simulink model "QAM16_NDATED_DDPED_2023b"  (R2023b)
settings: Solver=ode45  StartTime=0  StopTime=3200  RelTol=1e-3  EnableMultiTasking=on
PreLoadFcn:
  | SNR=30;                          % Signal-to-noise ratio
  | M=16;                             % No. QAM symbols
  | m=4;                               % log2(M) bits/symbol
  | T =  0.1;                          % Symbol period
  | Tc = T/10;                       % Carrier period
  | deltaf = 3e-3*(1/T);          % Frequency error
  | Tr = T+100e-6*T;            % Receiver clock
  | alpha = 0.25;                   % Rolloff factor
  | 
  | b3 = [1/6 -1/2  1/2 -1/6];
  | b2 = [1/2 -1    1/2  0];
  | b1 = [1/3  1/2 -1    1/6];
  | b0 = [0    1    0    0];
  | 
  | warning off all
values from neighbouring files (symbols this model uses):
  seed = input('Enter the last five digits of your student ID: ')    [run_OFDM_2011b.m]    (also in run_OFDM_2024b.m; run_RAKE_Rayleigh_2021b.m = input('Enter your student ID: '); run_RAKE_Rayleigh_2024b.m = input('Enter your student ID: '))
undefined symbols (not defined in the file or in its folder): dfilt, doppler, gcbh, QAM, rcfiltgaincompat
libraries: dspobslib x7, commfilt2 x4, dspfdesign x3, commdigbbndam3 x3, commchan3 x2, commrandsrc2 x1
settings Model: Creator=professor  LastModifiedBy=14083
settings SolverCC: AlgebraicLoopSolver=TrustRegion
settings DataIOCC: LimitDataPoints=on  SaveFormat=Array  SignalLoggingSaveFormat=ModelDataLogs  ReturnWorkspaceOutputs=off
settings OptimizationCC: ExpressionDepthLimit=2147483647  InitFltsAndDblsToZero=on  LifeSpan=inf
settings DebuggingCC: AlgebraicLoopMsg=none  SaveWithParameterizedLinksMsg=none  UnderspecifiedInitializationDetection=Classic  MergeDetectMultiDrivingBlocksExec=none  SolverPrmCheckMsg=warning  MultiTaskDSMMsg=warning  MultiTaskCondExecSysMsg=none  FcnCallInpInsideContextMsg=warning  UnconnectedInputMsg=warning  UnconnectedOutputMsg=warning  UnconnectedLineMsg=warning  StateNameClashWarn=warning  SFUnexpectedBacktrackingDiag=warning  SFNoUnconditionalDefaultTransitionDiag=warning  SFExecutionAtInitializationDiag=none  ArithmeticOperatorsInVariantConditions=warning
settings HardwareCC: ProdBitPerPointer=32  ProdBitPerSizeT=32  ProdBitPerPtrDiffT=32  ProdLargestAtomicFloat=None  ProdIntDivRoundTo=Undefined  ProdEndianess=Unspecified  ProdWordSize=32  ProdHWDeviceType=32-bit Generic
settings ModelReferenceCC: EnableRefExpFcnMdlSchedulingChecks=on  PropagateSignalLabelsOutOfModel=off
settings SFSimCC: SimUseLocalCustomCode=off  CustomCodeUndefinedFunction=UseInterfaceOnly
settings RTWCC: RTWUseLocalCustomCode=off
settings CodeAppCC: StateflowObjectComments=on
settings GRTTargetCC: TargetFcnLib=ansi_tfl_tmw.mat  TargetLangStandard=C89/C90 (ANSI)  CombineOutputUpdateFcns=off  GRTInterface=on
settings ConfigComp: CovMetricSettings=dw  CovSaveCumulativeToWorkspaceVar=on  CovSaveSingleToWorkspaceVar=on  CovExternalEMLEnable=off

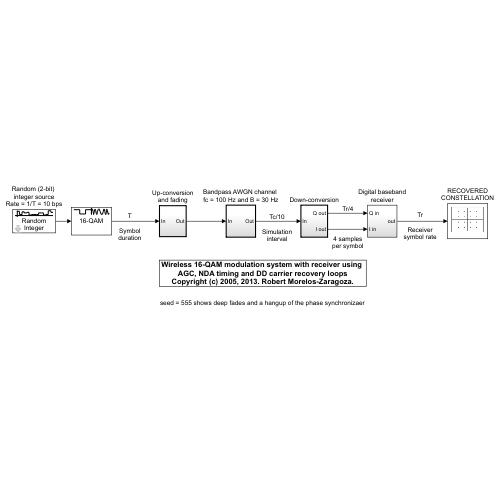
[thumbnail: Simulink's stored preview of the top-level diagram]
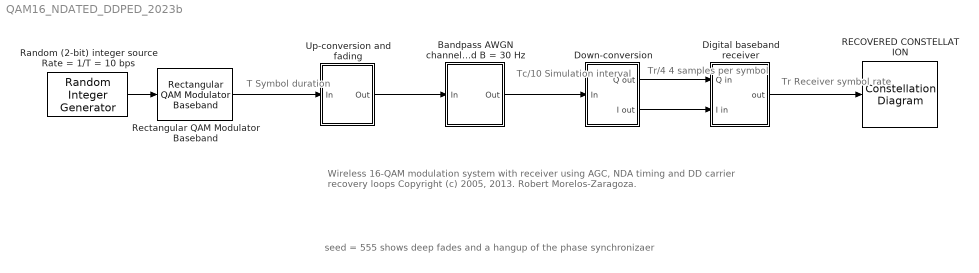
== system QAM16_NDATED_DDPED_2023b ==
  note: seed = 555 shows deep fades and a hangup of the phase synchronizaer
  note: Wireless 16-QAM modulation system with receiver using
      | AGC, NDA timing and DD carrier recovery loops
      | Copyright (c) 2005, 2013. Robert Morelos-Zaragoza.
  note: Tc/10
      |
      | Simulation
      | interval
  note: T
      |
      | Symbol
      | duration
  note: Tr/4
      |
      |
      |
      | 4 samples
      | per symbol
  note: Tr
      |
      | Receiver
      | symbol rate
  Bandpass AWGN channel fc = 100 Hz and B = 30 Hz : Subsystem  TreatAsAtomicUnit=on
  Digital baseband receiver : Subsystem
  Down-conversion : Subsystem  TreatAsAtomicUnit=on
  RECOVERED CONSTELLATION : ConstellationDiagram  Tag=ScatterPlot  WindowPosition=[323.000000,481.000000,326.000000,350.000000,]  Visible=on  ScopeFrameLocation=window  SymbolsToDisplaySource=Property  SymbolsToDisplay=150  ReferenceConstellation=16-QAM  Title=RECOVERED CONSTELLATION  XLimits=[-2.76,2.76]  YLimits=[-2.5 2.5]  DefaultConfigurationName=comm.scopes.ConstellationDiagramBlockCfg
  Random (2-bit) integer source Rate = 1/T = 10 bps : commrandsrc2/Random Integer Generator  mul=M  seed=seed  Ts=T  frameBased=off  sampPerFrame=1  orient=off  outDataType=double
  Rectangular QAM Modulator Baseband : commdigbbndam3/Rectangular QAM Modulator Baseband  M=M  InType=Integer  Enc=Gray  Mapping=[0:15]  PowType=Average Power  MinDist=2  AvgPow=1  PeakPow=1  Ph=0  outDtype=double  outWordLen=16  outUDDataType=sfix(16)  outFracLenMode=Best precision  outFracLen=15  outDataTypeStr=double  outLastDataTypeStr=double
  Up-conversion and fading : Subsystem  TreatAsAtomicUnit=on
  wires:
  Bandpass AWGN channel fc = 100 Hz and B = 30 Hz/1(Out) -> Down-conversion/1(In)
  Down-conversion/1(Q out) -> Digital baseband receiver/1(Q in)
  Down-conversion/2(I out) -> Digital baseband receiver/2(I in)
  Digital baseband receiver/1(out) -> RECOVERED CONSTELLATION/1
  Rectangular QAM Modulator Baseband/1 -> Up-conversion and fading/1(In)
  Random (2-bit) integer source Rate = 1/T = 10 bps/1 -> Rectangular QAM Modulator Baseband/1
  Up-conversion and fading/1(Out) -> Bandpass AWGN channel fc = 100 Hz and B = 30 Hz/1(In)

== system QAM16_NDATED_DDPED_2023b/Bandpass AWGN channel fc = 100 Hz and B = 30 Hz ==
  note: Bandpass AWGN channel
      |
      | Robert Morelos-Zaragoza
      | San Jose State University
      | Copyright (c) 2005
  In : Inport
  AWGN Channel : commchan3/AWGN Channel  LegacyMode=on  NoiseMethod="Signal to noise ratio  (SNR)"  noiseMode="Signal to noise ratio  (Eb/No)"  EbNo=SNR  EsNo=15  SNR=10  BitsPerSymbol=2  SignalPower=1  SamplesPerSymbol=1  SymbolPeriod=T/4  VarianceSource=Parameter  Variance=1  RandomStream=Global stream  Seed=13357  SimulateUsing=Code generation
  "Channel Hc(f) fc=100, B=30" : dspfdesign/Analog Filter Design  method=Chebyshev I  filttype=Bandpass  N=20  Wlo=2*pi*85  Whi=2*pi*115  Rp=0.5  Rs=30
  Tc/10 Simulation interval : ZeroOrderHold  SampleTime=Tc/10
  Out : Outport
  wires:
  "Channel Hc(f) fc=100, B=30"/1 -> Tc/10 Simulation interval/1
  AWGN Channel/1 -> Out/1
  In/1 -> "Channel Hc(f) fc=100, B=30"/1
  Tc/10 Simulation interval/1 -> AWGN Channel/1

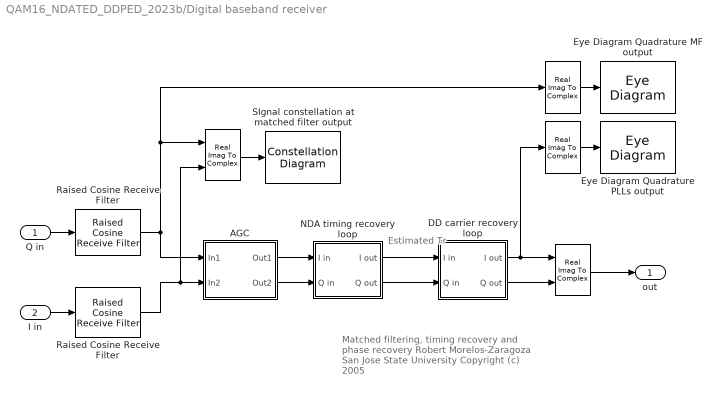
== system QAM16_NDATED_DDPED_2023b/Digital baseband receiver ==
  note: Estimated
      | Tr
  note: Matched filtering, timing recovery
      | and phase recovery
      |
      | Robert Morelos-Zaragoza
      | San Jose State University
      | Copyright (c) 2005
  Q in : Inport
  I in : Inport  Port=2
  " " : RealImagToComplex  Input=Real  SampleTime=Tr/4
  "    " : RealImagToComplex  SampleTime=Tr/4
  "       " : RealImagToComplex  Input=Real  SampleTime=Tr/4
  "           " : RealImagToComplex  SampleTime=Tr
  AGC : Subsystem  TreatAsAtomicUnit=on
  DD carrier recovery loop : Subsystem
  Eye Diagram Quadrature MF output : EyeDiagram  Tag=EyeDiagram
  Eye Diagram Quadrature PLLs output : EyeDiagram  Tag=EyeDiagram
  NDA timing recovery loop : Subsystem
  Raised Cosine Receive Filter : commfilt2/Raised Cosine Receive Filter  filtType=Square root  R=alpha  filtSpan=2*(4)  N=4  downFactor=1  downOffset=0  filterGain=(1/2)*rcfiltgaincompat(gcbh)  InputProcessing=Columns as channels (frame based)  RateOptions=Enforce single-rate processing  framing=Mute  checkCoeff=off  variableName=rcRxFilt  currentFiltSpan=2*(4)  D=4  inputOffset=0  sampMode=Mute  saveAsFlag=0  rateMode=Downsampling  checkGain=User-specified  launchFVT=off  roundingMode=Floor  overflowMode=off  coeffDataTypeStr=Inherit: Same word length as input  coeffMin=[]  coeffMax=[]  coeffLastDataTypeStr=Inherit: Same word length as input  accumDataTypeStr=Inherit: Same as product output  accumLastDataTypeStr=Inherit: Same as product output  outputDataTypeStr=Inherit: Same as accumulator  outputMin=[]  outputMax=[]  outputLastDataTypeStr=Inherit: Same as accumulator
  "Raised Cosine Receive Filter " : commfilt2/Raised Cosine Receive Filter  filtType=Square root  R=alpha  filtSpan=2*(4)  N=4  downFactor=1  downOffset=0  filterGain=(1/2)*rcfiltgaincompat(gcbh)  InputProcessing=Columns as channels (frame based)  RateOptions=Enforce single-rate processing  framing=Mute  checkCoeff=off  variableName=rcRxFilt1  currentFiltSpan=2*(4)  D=4  inputOffset=0  sampMode=Mute  saveAsFlag=0  rateMode=Downsampling  checkGain=User-specified  launchFVT=off  roundingMode=Floor  overflowMode=off  coeffDataTypeStr=Inherit: Same word length as input  coeffMin=[]  coeffMax=[]  coeffLastDataTypeStr=Inherit: Same word length as input  accumDataTypeStr=Inherit: Same as product output  accumLastDataTypeStr=Inherit: Same as product output  outputDataTypeStr=Inherit: Same as accumulator  outputMin=[]  outputMax=[]  outputLastDataTypeStr=Inherit: Same as accumulator
  SIgnal constellation at matched filter output : ConstellationDiagram  Tag=ScatterPlot  WindowPosition=[-1.000000,481.000000,322.000000,351.000000,]  Visible=on  ScopeFrameLocation=window  SamplesPerSymbol=4  SampleOffset=1  SymbolsToDisplaySource=Property  SymbolsToDisplay=150  ReferenceConstellation=16-QAM  Title=MF OUTPUT CONSTELLATION  XLimits=[-2.71,2.71]  YLimits=[-2.5 2.5]  DefaultConfigurationName=comm.scopes.ConstellationDiagramBlockCfg
  out : Outport
  wires:
  Q in/1 -> Raised Cosine Receive Filter/1
  I in/1 -> "Raised Cosine Receive Filter "/1
  Raised Cosine Receive Filter/1 -> "    "/1, " "/1, AGC/1(In1)
  "    "/1 -> SIgnal constellation at matched filter output/1
  DD carrier recovery loop/1(I out) -> "           "/1, "       "/1
  DD carrier recovery loop/2(Q out) -> "           "/2
  "           "/1 -> out/1
  NDA timing recovery loop/1(I out) -> DD carrier recovery loop/1(I in)
  NDA timing recovery loop/2(Q out) -> DD carrier recovery loop/2(Q in)
  " "/1 -> Eye Diagram Quadrature MF output/1
  "       "/1 -> Eye Diagram Quadrature PLLs output/1
  "Raised Cosine Receive Filter "/1 -> "    "/2, AGC/2(In2)
  AGC/1(Out1) -> NDA timing recovery loop/1(I in)
  AGC/2(Out2) -> NDA timing recovery loop/2(Q in)

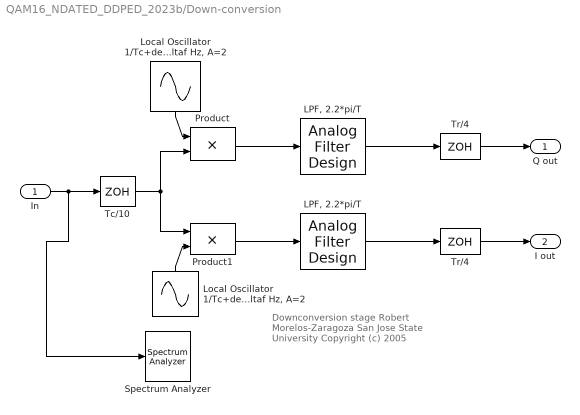
== system QAM16_NDATED_DDPED_2023b/Down-conversion ==
  note: Downconversion stage
      |
      | Robert Morelos-Zaragoza
      | San Jose State University
      | Copyright (c) 2005
  In : Inport
  " LPF, 2.2*pi/T " : dspfdesign/Analog Filter Design  method=Butterworth  filttype=Lowpass  N=8  Wlo=2.2*pi/T  Whi=80  Rp=2  Rs=40
  "LPF, 2.2*pi/T" : dspfdesign/Analog Filter Design  method=Butterworth  filttype=Lowpass  N=8  Wlo=2.2*pi/T  Whi=80  Rp=2  Rs=40
  "Local Oscillator 1/Tc+deltaf Hz, A=2 " : Sin  Amplitude=2  Frequency=2*pi/Tc+deltaf  SampleTime=Tc/10
  "Local Oscillator 1/Tc+deltaf Hz, A=2    " : Sin  Amplitude=2  Frequency=2*pi/Tc+deltaf  Phase=pi/2  SampleTime=Tc/10
  Product : Product  InputSameDT=on  SaturateOnIntegerOverflow=on  OutDataTypeStr=Inherit: Same as first input
  Product1 : Product  InputSameDT=on  SaturateOnIntegerOverflow=on  OutDataTypeStr=Inherit: Same as first input
  Spectrum Analyzer : SpectrumAnalyzer  WindowPosition=[1055.000000,511.000000,477.000000,319.000000,]  Visible=on  ScopeFrameLocation=window  AxesScaling=Manual  Span=1000  StartFrequency=-500  StopFrequency=500  YLimits=[-30,30]
  Tc/10 : ZeroOrderHold  SampleTime=Tc/10
  Tr/4 : ZeroOrderHold  SampleTime=Tr/4
  "Tr/4 " : ZeroOrderHold  SampleTime=Tr/4
  Q out : Outport
  I out : Outport  Port=2
  wires:
  "Local Oscillator 1/Tc+deltaf Hz, A=2    "/1 -> Product1/2
  "LPF, 2.2*pi/T"/1 -> Tr/4/1
  "Local Oscillator 1/Tc+deltaf Hz, A=2 "/1 -> Product/1
  Product/1 -> "LPF, 2.2*pi/T"/1
  " LPF, 2.2*pi/T "/1 -> "Tr/4 "/1
  Product1/1 -> " LPF, 2.2*pi/T "/1
  In/1 -> Spectrum Analyzer/1, Tc/10/1
  Tr/4/1 -> Q out/1
  "Tr/4 "/1 -> I out/1
  Tc/10/1 -> Product/2, Product1/1

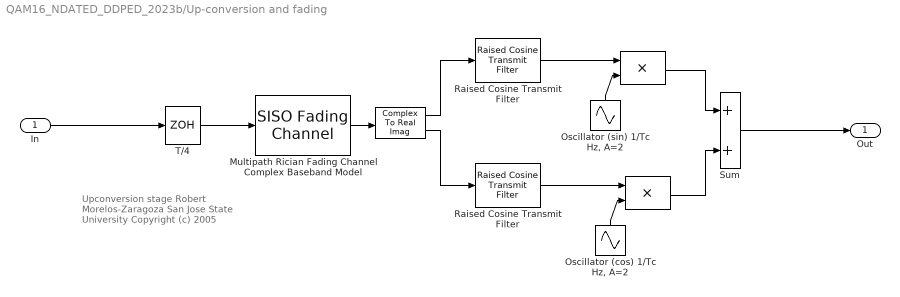
== system QAM16_NDATED_DDPED_2023b/Up-conversion and fading ==
  note: Upconversion stage
      |
      | Robert Morelos-Zaragoza
      | San Jose State University
      | Copyright (c) 2005
  In : Inport
  " " : ComplexToRealImag
  "  " : Product  InputSameDT=on  SaturateOnIntegerOverflow=on  OutDataTypeStr=Inherit: Same as first input
  "   " : Product  InputSameDT=on  SaturateOnIntegerOverflow=on  OutDataTypeStr=Inherit: Same as first input
  Multipath Rician Fading Channel Complex Baseband Model : commchan3/SISO Fading Channel  InheritSampleRate=on  SampleRate=1  PathDelays=0  AveragePathGains=-3  NormalizePathGains=on  FadingDistribution=Rician  KFactor=1  DirectPathDopplerShift=.001  DirectPathInitialPhase=0  MaximumDopplerShift=7e-5  DopplerSpectrum=doppler('Jakes')  RandomStream=mt19937ar with seed  Seed=mod(seed,100)  PathGainsOutputPort=off  ChannelFilterDelayOutputPort=off  SimulateUsing=Interpreted execution  Visualization=Off  PathsForDopplerDisplay=1  SamplesToDisplay=25%
  "Oscillator (cos) 1/Tc Hz, A=2" : Sin  Amplitude=2  Frequency=2*pi/Tc  Phase=pi/2  SampleTime=0
  "Oscillator (sin) 1/Tc Hz, A=2 " : Sin  Amplitude=2  Frequency=2*pi/Tc  SampleTime=0
  Raised Cosine Transmit Filter : commfilt2/Raised Cosine Transmit Filter  filtType=Square root  R=alpha  filtSpan=2*(4)  N=4  filterGain=rcfiltgaincompat(gcbh)  InputProcessing=Columns as channels (frame based)  RateOptions=Allow multirate processing  framing=Mute  checkCoeff=off  variableName=rcTxFilt  checkGain=Normalized  sampMode=Mute  saveAsFlag=0  currentFiltSpan=2*(4)  D=4  launchFVT=off  roundingMode=Floor  overflowMode=off  coeffDataTypeStr=Inherit: Same word length as input  coeffMin=[]  coeffMax=[]  coeffLastDataTypeStr=Inherit: Same word length as input  outputDataTypeStr=Inherit: Same as accumulator  outputMin=[]  outputMax=[]  outputLastDataTypeStr=Inherit: Same as accumulator
  "Raised Cosine Transmit Filter " : commfilt2/Raised Cosine Transmit Filter  filtType=Square root  R=alpha  filtSpan=2*(4)  N=4  filterGain=rcfiltgaincompat(gcbh)  InputProcessing=Columns as channels (frame based)  RateOptions=Allow multirate processing  framing=Mute  checkCoeff=off  variableName=rcTxFilt1  checkGain=Normalized  sampMode=Mute  saveAsFlag=0  currentFiltSpan=2*(4)  D=4  launchFVT=off  roundingMode=Floor  overflowMode=off  coeffDataTypeStr=Inherit: Same word length as input  coeffMin=[]  coeffMax=[]  coeffLastDataTypeStr=Inherit: Same word length as input  outputDataTypeStr=Inherit: Same as accumulator  outputMin=[]  outputMax=[]  outputLastDataTypeStr=Inherit: Same as accumulator
  Sum : Sum  InputSameDT=on  SaturateOnIntegerOverflow=on  OutDataTypeStr=Inherit: Same as first input
  T/4 : ZeroOrderHold  SampleTime=T/4
  Out : Outport
  wires:
  T/4/1 -> Multipath Rician Fading Channel Complex Baseband Model/1
  In/1 -> T/4/1
  Raised Cosine Transmit Filter/1 -> "  "/1
  "Raised Cosine Transmit Filter "/1 -> "   "/1
  "Oscillator (sin) 1/Tc Hz, A=2 "/1 -> "  "/2
  "Oscillator (cos) 1/Tc Hz, A=2"/1 -> "   "/2
  "  "/1 -> Sum/1
  "   "/1 -> Sum/2
  Sum/1 -> Out/1
  " "/1 -> Raised Cosine Transmit Filter/1
  " "/2 -> "Raised Cosine Transmit Filter "/1
  Multipath Rician Fading Channel Complex Baseband Model/1 -> " "/1

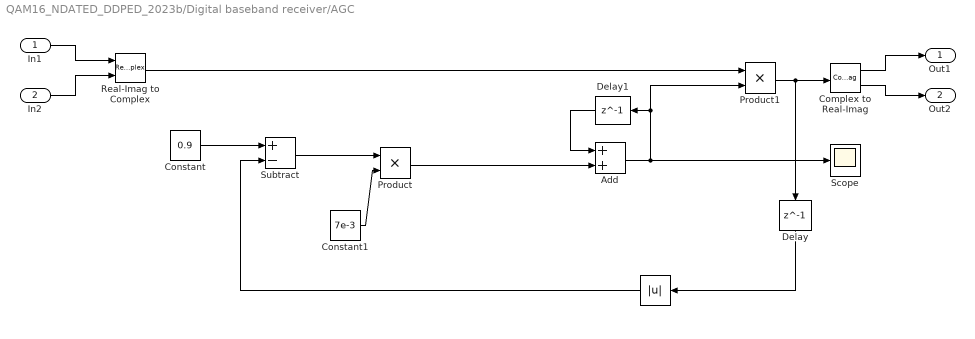
== system QAM16_NDATED_DDPED_2023b/Digital baseband receiver/AGC ==
  In1 : Inport
  In2 : Inport  Port=2
  " " : Abs  SaturateOnIntegerOverflow=off
  Add : Sum
  Complex to Real-Imag : ComplexToRealImag
  Constant : Constant  Value=0.9
  Constant1 : Constant  Value=7e-3
  Delay : Delay  DelayLength=1  InitialCondition=0  InputProcessing=Columns as channels (frame based)
  Delay1 : Delay  DelayLength=1  InitialCondition=1  InputProcessing=Columns as channels (frame based)
  Product : Product  RndMeth=Zero
  Product1 : Product  RndMeth=Zero
  Real-Imag to Complex : RealImagToComplex
  Scope : Scope
  Subtract : Sum  Inputs=+-
  Out1 : Outport
  Out2 : Outport  Port=2
  wires:
  Subtract/1 -> Product/1
  Constant1/1 -> Product/2
  In1/1 -> Real-Imag to Complex/1
  In2/1 -> Real-Imag to Complex/2
  Real-Imag to Complex/1 -> Product1/1
  Complex to Real-Imag/1 -> Out1/1
  Complex to Real-Imag/2 -> Out2/1
  Product1/1 -> Delay/1, Complex to Real-Imag/1
  Delay/1 -> " "/1
  Product/1 -> Add/2
  Add/1 -> Scope/1, Product1/2, Delay1/1
  Delay1/1 -> Add/1
  Constant/1 -> Subtract/1
  " "/1 -> Subtract/2

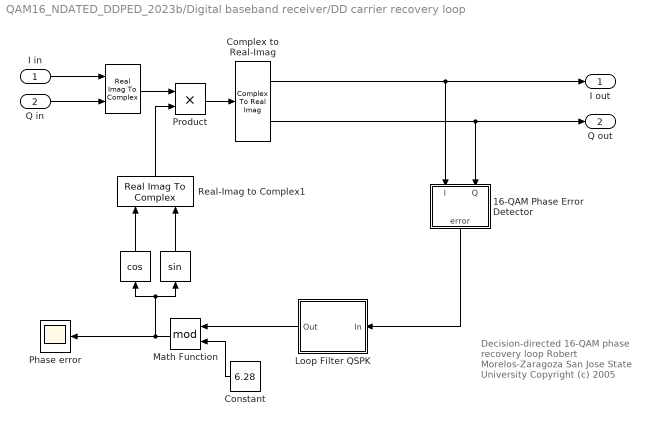
== system QAM16_NDATED_DDPED_2023b/Digital baseband receiver/DD carrier recovery loop ==
  note: Decision-directed 16-QAM
      | phase recovery loop
      |
      | Robert Morelos-Zaragoza
      | San Jose State University
      | Copyright (c) 2005
  I in : Inport
  Q in : Inport  Port=2
  " " : Trigonometry  OutputSignalType=real
  "   " : Trigonometry  Operator=cos  OutputSignalType=real
  "     " : RealImagToComplex  SampleTime=Tr
  "  16-QAM Phase Error Detector" : Subsystem
  Complex to Real-Imag : ComplexToRealImag
  Constant : Constant  Value=6.28  SampleTime=Tr
  Loop Filter QSPK : Subsystem
  Math Function : Math  Operator=mod  SignedPower=on  OutputSignalType=real  SampleTime=Tr
  Phase error : Scope
  Product : Product  InputSameDT=on  OutDataTypeStr=Inherit: Same as first input
  Real-Imag to Complex1 : RealImagToComplex
  I out : Outport
  Q out : Outport  Port=2
  wires:
  Real-Imag to Complex1/1 -> Product/2
  "   "/1 -> Real-Imag to Complex1/1
  " "/1 -> Real-Imag to Complex1/2
  Product/1 -> Complex to Real-Imag/1
  Complex to Real-Imag/1 -> I out/1, "  16-QAM Phase Error Detector"/1(I)
  Complex to Real-Imag/2 -> Q out/1, "  16-QAM Phase Error Detector"/2(Q)
  Loop Filter QSPK/1(Out) -> Math Function/1
  Constant/1 -> Math Function/2
  Math Function/1 -> " "/1, "   "/1, Phase error/1
  I in/1 -> "     "/1
  Q in/1 -> "     "/2
  "     "/1 -> Product/1
  "  16-QAM Phase Error Detector"/1(error) -> Loop Filter QSPK/1(In)

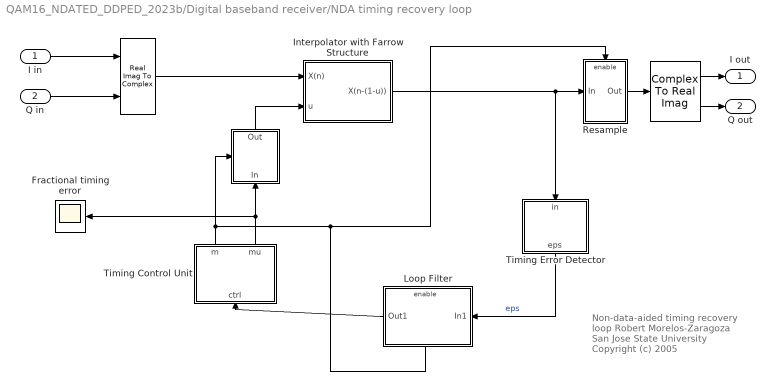
== system QAM16_NDATED_DDPED_2023b/Digital baseband receiver/NDA timing recovery loop ==
  note: Non-data-aided timing
      | recovery loop
      |
      | Robert Morelos-Zaragoza
      | San Jose State University
      | Copyright (c) 2005
  I in : Inport
  Q in : Inport  Port=2
  " " : ComplexToRealImag
  "     " : RealImagToComplex  SampleTime=Tr/4
  "         " : Subsystem  TreatAsAtomicUnit=on
  "  Timing Error Detector " : Subsystem
  Fractional timing error : Scope
  "Interpolator with Farrow Structure " : Subsystem
  "Loop Filter " : Subsystem  TreatAsAtomicUnit=on
  Resample : Subsystem  TreatAsAtomicUnit=on
  "Timing Control Unit   " : Subsystem
  I out : Outport
  Q out : Outport  Port=2
  wires:
  I in/1 -> "     "/1
  Q in/1 -> "     "/2
  "Interpolator with Farrow Structure "/1(X(n-(1-u))) -> Resample/1(In), "  Timing Error Detector "/1(in)
  "     "/1 -> "Interpolator with Farrow Structure "/1(X(n))
  "  Timing Error Detector "/1(eps) -> "Loop Filter "/1(In1)  "eps"
  " "/1 -> I out/1
  " "/2 -> Q out/1
  Resample/1(Out) -> " "/1
  "Loop Filter "/1(Out1) -> "Timing Control Unit   "/1(ctrl)
  "Timing Control Unit   "/2(mu) -> "         "/1(In), Fractional timing error/1
  "         "/1(Out) -> "Interpolator with Farrow Structure "/2(u)
  "Timing Control Unit   "/1(m) -> "         "/Enable, Resample/Enable, "Loop Filter "/Enable

== system QAM16_NDATED_DDPED_2023b/Digital baseband receiver/DD carrier recovery loop/  16-QAM Phase Error Detector ==
  I : Inport
  Q : Inport  Port=2
  Complex to Real-Imag : ComplexToRealImag  Output=Imag
  Math Function : Math  Operator=hermitian  SignedPower=on
  Product : Product  InputSameDT=on  RndMeth=Zero  SaturateOnIntegerOverflow=on  OutDataTypeStr=Inherit: Same as first input
  Real-Imag to Complex : RealImagToComplex
  Rectangular QAM Demodulator Baseband : commdigbbndam3/Rectangular QAM Demodulator Baseband  M=M  OutType=Integer  DecType=Hard decision  VarSource=Dialog  Variance=1  Dec=Gray  Mapping=[0:15]  PowType=Average Power  MinDist=2  AvgPow=1  PeakPow=1  Ph=0  outDtype1=Inherit via internal rule  outDtype2=Inherit via internal rule  derotateFactorWordLen=16  derotateFactorDataTypeStr=Inherit: Same word length as input  derotateFactorLastDataTypeStr=Inherit: Same word length as input  denormFactorWordLen=16  denormFactorDataTypeStr=Inherit: Same word length as input  denormFactorLastDataTypeStr=Inherit: Same word length as input  prodOutWordLen=32  prodOutOverflowMode=Wrap  prodOutRoundingMode=Floor  prodOutOvFlMode=off  prodOutOvFlModeLastStrValue=off  sumWordLen=32
  Rectangular QAM Modulator Baseband : commdigbbndam3/Rectangular QAM Modulator Baseband  M=M  InType=Integer  Enc=Gray  Mapping=[0:15]  PowType=Average Power  MinDist=2  AvgPow=1  PeakPow=1  Ph=0  outDtype=double  outWordLen=16  outUDDataType=sfix(16)  outFracLenMode=Best precision  outFracLen=15  outDataTypeStr=double  outLastDataTypeStr=double
  error : Outport
  wires:
  Rectangular QAM Demodulator Baseband/1 -> Rectangular QAM Modulator Baseband/1
  Real-Imag to Complex/1 -> Rectangular QAM Demodulator Baseband/1, Product/1
  I/1 -> Real-Imag to Complex/1
  Q/1 -> Real-Imag to Complex/2
  Product/1 -> Complex to Real-Imag/1
  Complex to Real-Imag/1 -> error/1
  Rectangular QAM Modulator Baseband/1 -> Math Function/1
  Math Function/1 -> Product/2

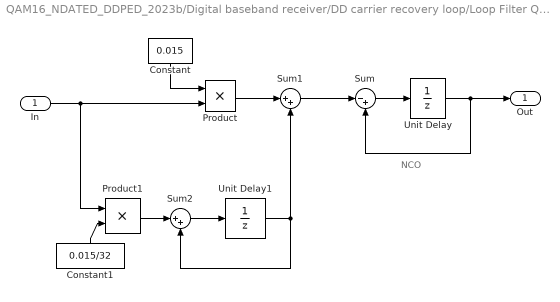
== system QAM16_NDATED_DDPED_2023b/Digital baseband receiver/DD carrier recovery loop/Loop Filter QSPK ==
  note: NCO
  In : Inport
  Constant : Constant  Value=0.015  SampleTime=Tr
  Constant1 : Constant  Value=0.015/32  SampleTime=Tr
  Product : Product  InputSameDT=on  SaturateOnIntegerOverflow=on  SampleTime=Tr  OutDataTypeStr=Inherit: Same as first input
  Product1 : Product  InputSameDT=on  SaturateOnIntegerOverflow=on  SampleTime=Tr  OutDataTypeStr=Inherit: Same as first input
  Sum : Sum  Inputs=|-+  InputSameDT=on  SaturateOnIntegerOverflow=on  OutDataTypeStr=Inherit: Same as first input
  Sum1 : Sum  Inputs=|++  InputSameDT=on  SaturateOnIntegerOverflow=on  OutDataTypeStr=Inherit: Same as first input
  Sum2 : Sum  Inputs=|++  InputSameDT=on  SaturateOnIntegerOverflow=on  OutDataTypeStr=Inherit: Same as first input
  Unit Delay : UnitDelay  SampleTime=Tr  HasFrameUpgradeWarning=on
  Unit Delay1 : UnitDelay  SampleTime=Tr  HasFrameUpgradeWarning=on
  Out : Outport
  wires:
  Product/1 -> Sum1/1
  Constant1/1 -> Product1/2
  Sum/1 -> Unit Delay/1
  Unit Delay/1 -> Out/1, Sum/2
  Constant/1 -> Product/1
  In/1 -> Product/2, Product1/1
  Product1/1 -> Sum2/1
  Sum2/1 -> Unit Delay1/1
  Unit Delay1/1 -> Sum1/2, Sum2/2
  Sum1/1 -> Sum/1

== system QAM16_NDATED_DDPED_2023b/Digital baseband receiver/NDA timing recovery loop/          ==
  In : Inport
  Enable : EnablePort
  Out : Outport
  wires:
  In/1 -> Out/1

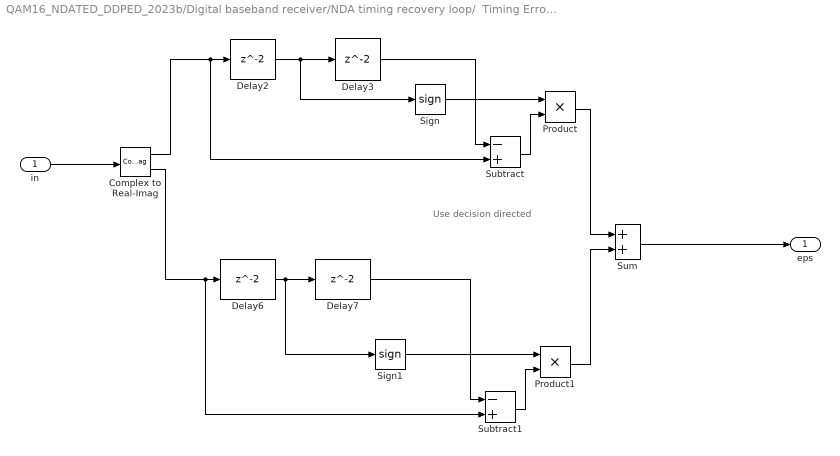
== system QAM16_NDATED_DDPED_2023b/Digital baseband receiver/NDA timing recovery loop/  Timing Error Detector  ==
  note: Use decision directed
  in : Inport
  Complex to Real-Imag : ComplexToRealImag
  Delay{2..3,6..7} (4 alike) : Delay  InitialCondition=0  InputProcessing=Columns as channels (frame based)
  Product : Product  RndMeth=Zero
  Product1 : Product  RndMeth=Zero
  Sign : Signum
  Sign1 : Signum
  Subtract : Sum  Inputs=-+
  Subtract1 : Sum  Inputs=-+
  Sum : Sum
  eps : Outport
  wires:
  Delay3/1 -> Subtract/1
  Delay7/1 -> Subtract1/1
  in/1 -> Complex to Real-Imag/1
  Complex to Real-Imag/1 -> Delay2/1, Subtract/2
  Complex to Real-Imag/2 -> Delay6/1, Subtract1/2
  Sum/1 -> eps/1
  Subtract1/1 -> Product1/2
  Product1/1 -> Sum/2
  Subtract/1 -> Product/2
  Product/1 -> Sum/1
  Delay2/1 -> Delay3/1, Sign/1
  Delay6/1 -> Delay7/1, Sign1/1
  Sign/1 -> Product/1
  Sign1/1 -> Product1/1

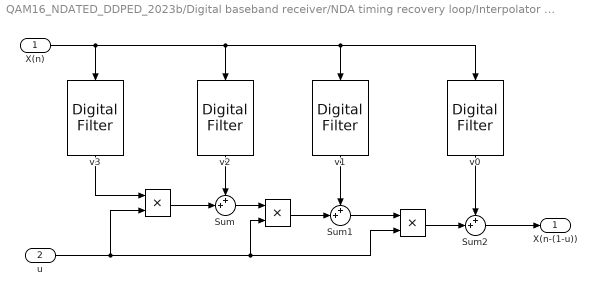
== system QAM16_NDATED_DDPED_2023b/Digital baseband receiver/NDA timing recovery loop/Interpolator with Farrow Structure  ==
  X(n) : Inport
  u : Inport  Port=2
  " " : Product  SaturateOnIntegerOverflow=on  OutDataTypeStr=Inherit: Same as first input
  "  " : Product  SaturateOnIntegerOverflow=on  OutDataTypeStr=Inherit: Same as first input
  "   " : Product  SaturateOnIntegerOverflow=on  OutDataTypeStr=Inherit: Same as first input
  Sum : Sum  Inputs=++|  SaturateOnIntegerOverflow=on
  Sum1 : Sum  Inputs=++|  SaturateOnIntegerOverflow=on
  Sum2 : Sum  Inputs=++|  SaturateOnIntegerOverflow=on
  v0 : dspobslib/Digital Filter  TypePopup=FIR (all zeros)  IIRFiltStruct=Direct form II transposed  AllPoleFiltStruct=Direct form  FIRFiltStruct=Direct form  CoeffSource=Specify via dialog  NumCoeffs=b0  DenCoeffs=[1 0.1]  BiQuadCoeffs=[1 0.3 0.4 1 0.1 0.2]  LatticeCoeffs=[0.2 0.4]  denIgnore=on  FiltPerSampPopup=One filter per frame  IC=0  ICnum=0  ICden=0  roundingMode=Floor  overflowMode=off  ScaleValues=1  scaleValueFracLength=14  stageInFracLength=15  stageOutFracLength=15  FilterSource=Specify via dialog  dfiltObjectName=dfilt.dffir([1 2 1])  InputProcessing=Columns as channels (frame based)
  v1 : dspobslib/Digital Filter  TypePopup=FIR (all zeros)  IIRFiltStruct=Direct form II transposed  AllPoleFiltStruct=Direct form  FIRFiltStruct=Direct form  CoeffSource=Specify via dialog  NumCoeffs=b1  DenCoeffs=[1 0.1]  BiQuadCoeffs=[1 0.3 0.4 1 0.1 0.2]  LatticeCoeffs=[0.2 0.4]  denIgnore=on  FiltPerSampPopup=One filter per frame  IC=0  ICnum=0  ICden=0  roundingMode=Floor  overflowMode=off  ScaleValues=1  scaleValueFracLength=14  stageInFracLength=15  stageOutFracLength=15  FilterSource=Specify via dialog  dfiltObjectName=dfilt.dffir([1 2 1])  InputProcessing=Columns as channels (frame based)
  v2 : dspobslib/Digital Filter  TypePopup=FIR (all zeros)  IIRFiltStruct=Direct form II transposed  AllPoleFiltStruct=Direct form  FIRFiltStruct=Direct form  CoeffSource=Specify via dialog  NumCoeffs=b2  DenCoeffs=[1 0.1]  BiQuadCoeffs=[1 0.3 0.4 1 0.1 0.2]  LatticeCoeffs=[0.2 0.4]  denIgnore=on  FiltPerSampPopup=One filter per frame  IC=0  ICnum=0  ICden=0  roundingMode=Floor  overflowMode=off  ScaleValues=1  scaleValueFracLength=14  stageInFracLength=15  stageOutFracLength=15  FilterSource=Specify via dialog  dfiltObjectName=dfilt.dffir([1 2 1])  InputProcessing=Columns as channels (frame based)
  v3 : dspobslib/Digital Filter  TypePopup=FIR (all zeros)  IIRFiltStruct=Direct form II transposed  AllPoleFiltStruct=Direct form  FIRFiltStruct=Direct form  CoeffSource=Specify via dialog  NumCoeffs=b3  DenCoeffs=[1 0.1]  BiQuadCoeffs=[1 0.3 0.4 1 0.1 0.2]  LatticeCoeffs=[0.2 0.4]  denIgnore=on  FiltPerSampPopup=One filter per frame  IC=0  ICnum=0  ICden=0  roundingMode=Floor  overflowMode=off  ScaleValues=1  scaleValueFracLength=14  stageInFracLength=15  stageOutFracLength=15  FilterSource=Specify via dialog  dfiltObjectName=dfilt.dffir([1 2 1])  InputProcessing=Columns as channels (frame based)
  X(n-(1-u)) : Outport
  wires:
  Sum2/1 -> X(n-(1-u))/1
  u/1 -> "   "/2, "  "/2, " "/2
  X(n)/1 -> v3/1, v2/1, v1/1, v0/1
  v0/1 -> Sum2/1
  v1/1 -> Sum1/1
  v2/1 -> Sum/1
  v3/1 -> " "/1
  " "/1 -> Sum/2
  Sum/1 -> "  "/1
  "  "/1 -> Sum1/2
  Sum1/1 -> "   "/1
  "   "/1 -> Sum2/2

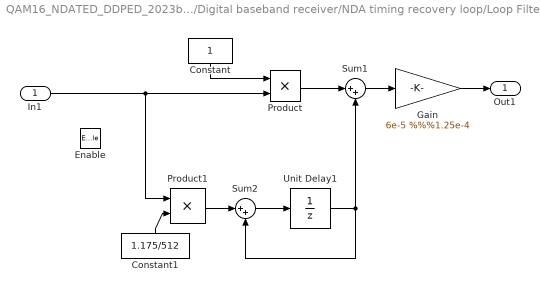
== system QAM16_NDATED_DDPED_2023b/Digital baseband receiver/NDA timing recovery loop/Loop Filter  ==
  In1 : Inport
  Enable : EnablePort
  Constant : Constant  SampleTime=Tr/4
  Constant1 : Constant  Value=1.175/512  SampleTime=Tr/4
  Gain : Gain  Gain=6e-5 %%%1.25e-4
  Product : Product  InputSameDT=on  SaturateOnIntegerOverflow=on  OutDataTypeStr=Inherit: Same as first input
  Product1 : Product  InputSameDT=on  SaturateOnIntegerOverflow=on  OutDataTypeStr=Inherit: Same as first input
  Sum1 : Sum  Inputs=|++  InputSameDT=on  SaturateOnIntegerOverflow=on  OutDataTypeStr=Inherit: Same as first input
  Sum2 : Sum  Inputs=|++  InputSameDT=on  SaturateOnIntegerOverflow=on  OutDataTypeStr=Inherit: Same as first input
  Unit Delay1 : UnitDelay  SampleTime=-1  HasFrameUpgradeWarning=on
  Out1 : Outport
  wires:
  Product/1 -> Sum1/1
  Constant1/1 -> Product1/2
  Constant/1 -> Product/1
  In1/1 -> Product/2, Product1/1
  Product1/1 -> Sum2/1
  Sum2/1 -> Unit Delay1/1
  Unit Delay1/1 -> Sum1/2, Sum2/2
  Sum1/1 -> Gain/1
  Gain/1 -> Out1/1

== system QAM16_NDATED_DDPED_2023b/Digital baseband receiver/NDA timing recovery loop/Resample ==
  In : Inport
  Enable : EnablePort
  Out : Outport
  wires:
  In/1 -> Out/1

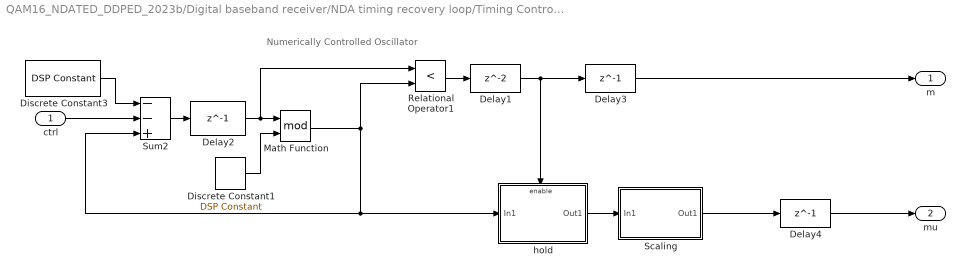
== system QAM16_NDATED_DDPED_2023b/Digital baseband receiver/NDA timing recovery loop/Timing Control Unit    ==
  note: Numerically Controlled Oscillator
  ctrl : Inport
  Delay1 : Delay  InitialCondition=0  InputProcessing=Columns as channels (frame based)
  Delay2 : Delay  DelayLength=1  InitialCondition=0  InputProcessing=Columns as channels (frame based)
  Delay3 : Delay  DelayLength=1  InitialCondition=0  InputProcessing=Columns as channels (frame based)
  Delay4 : Delay  DelayLength=1  InitialCondition=0  InputProcessing=Columns as channels (frame based)
  Discrete Constant1 : dspobslib/DSP Constant  Value=1  SampleMode=Discrete  discreteOutput=Sample-based (interpret vectors as 1-D)  continuousOutput=Sample-based  sampTime=Tr/4  framePeriod=Tr/4  dataType=Inherit via back propagation  isSigned=on  wordLen=16  udDataType=sfix(16)  fracBitsMode=Best precision  numFracBits=15  InterpretAs1D=on  Ts=Tr/4  FramebasedOutput=off
      settings: additionalParams=on
  Discrete Constant3 : dspobslib/DSP Constant  Value=1/4  SampleMode=Discrete  discreteOutput=Sample-based (interpret vectors as 1-D)  continuousOutput=Sample-based  sampTime=Tr/4  framePeriod=Tr/4  dataType=Inherit via back propagation  isSigned=on  wordLen=16  udDataType=sfix(16)  fracBitsMode=Best precision  numFracBits=15  InterpretAs1D=on  Ts=Tr/4  FramebasedOutput=off
      settings: additionalParams=on
  Math Function : Math  Operator=mod  SignedPower=on  SampleTime=Tr/4
  Relational Operator1 : RelationalOperator  Operator=<  OutDataTypeStr=boolean  SampleTime=Tr/4  InputSameDT=off
  Scaling : Subsystem
  Sum2 : Sum  Inputs=--+  InputSameDT=on  SaturateOnIntegerOverflow=on  SampleTime=Tr/4  OutDataTypeStr=Inherit: Same as first input
  hold : Subsystem  TreatAsAtomicUnit=on
  m : Outport
  mu : Outport  Port=2
  wires:
  Delay2/1 -> Math Function/1, Relational Operator1/1
  Discrete Constant1/1 -> Math Function/2
  Sum2/1 -> Delay2/1
  ctrl/1 -> Sum2/2
  Math Function/1 -> Relational Operator1/2, hold/1(In1), Sum2/3
  Relational Operator1/1 -> Delay1/1
  hold/1(Out1) -> Scaling/1(In1)
  Discrete Constant3/1 -> Sum2/1
  Delay3/1 -> m/1
  Scaling/1(Out1) -> Delay4/1
  Delay4/1 -> mu/1
  Delay1/1 -> hold/Enable, Delay3/1

== system QAM16_NDATED_DDPED_2023b/Digital baseband receiver/NDA timing recovery loop/Timing Control Unit   /Scaling ==
  In1 : Inport
  Add : Sum
  Discrete Constant1 : dspobslib/DSP Constant  Value=1  SampleMode=Discrete  discreteOutput=Sample-based (interpret vectors as 1-D)  continuousOutput=Sample-based  sampTime=Tr/4  framePeriod=Tr/4  dataType=Inherit via back propagation  isSigned=on  wordLen=16  udDataType=sfix(16)  fracBitsMode=Best precision  numFracBits=15  InterpretAs1D=on  Ts=Tr/4  FramebasedOutput=off
      settings: additionalParams=on
  Gain2 : Gain  Gain=4
  Math Function : Math  Operator=mod  SignedPower=on
  k5 : Constant  Value=-2  SampleTime=Tr/4
  Out1 : Outport
  wires:
  In1/1 -> Gain2/1
  k5/1 -> Add/2
  Gain2/1 -> Add/1
  Add/1 -> Math Function/1
  Math Function/1 -> Out1/1
  Discrete Constant1/1 -> Math Function/2

== system QAM16_NDATED_DDPED_2023b/Digital baseband receiver/NDA timing recovery loop/Timing Control Unit   /hold ==
  In1 : Inport
  Enable : EnablePort
  Out1 : Outport
  wires:
  In1/1 -> Out1/1
